simulink model "gui"  (R2012b)
settings: Solver=ode45  StartTime=0.0  StopTime=inf  RelTol=1e-3
undefined symbols (not defined in the file or in its folder): desired_torso_pitch, kd_lateral, kd_pitch, kd_sea_position, kd_sea_torque, ki_lateral, ki_sea_position, ki_sea_torque, kp_lateral, kp_pitch, kp_sea_position, kp_sea_torque, umich_kd1, umich_kd2, umich_kp1, umich_kp2, umich_sat_val1, umich_scuff1, umich_scuff2
libraries: simulink x20, xpclib x18
settings Model: Creator=wmartin  LastModifiedBy=wmartin

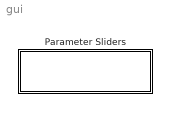
== system gui ==
  Parameter Sliders : Subsystem

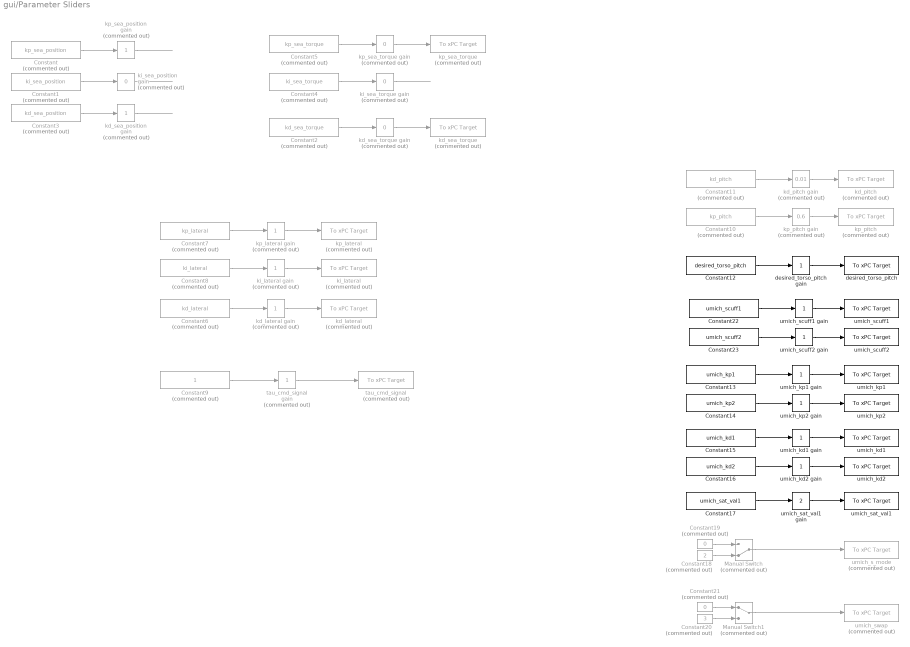
== system gui/Parameter Sliders ==
  Constant : Constant  Commented=on  Value=kp_sea_position
  Constant1 : Constant  Commented=on  Value=ki_sea_position
  Constant10 : Constant  Commented=on  Value=kp_pitch
  Constant11 : Constant  Commented=on  Value=kd_pitch
  Constant12 : Constant  Value=desired_torso_pitch
  Constant13 : Constant  Value=umich_kp1
  Constant14 : Constant  Value=umich_kp2
  Constant15 : Constant  Value=umich_kd1
  Constant16 : Constant  Value=umich_kd2
  Constant17 : Constant  Value=umich_sat_val1
  Constant18 : Constant  Commented=on  Value=2
  Constant19 : Constant  Commented=on  Value=0
  Constant2 : Constant  Commented=on  Value=kd_sea_torque
  Constant20 : Constant  Commented=on  Value=3
  Constant21 : Constant  Commented=on  Value=0
  Constant22 : Constant  Value=umich_scuff1
  Constant23 : Constant  Value=umich_scuff2
  Constant3 : Constant  Commented=on  Value=kd_sea_position
  Constant4 : Constant  Commented=on  Value=ki_sea_torque
  Constant5 : Constant  Commented=on  Value=kp_sea_torque
  Constant6 : Constant  Commented=on  Value=kd_lateral
  Constant7 : Constant  Commented=on  Value=kp_lateral
  Constant8 : Constant  Commented=on  Value=ki_lateral
  Constant9 : Constant  Commented=on
  Manual Switch : ManualSwitch  Commented=on  CurrentSetting=0
  Manual Switch1 : ManualSwitch  Commented=on
  desired_torso_pitch : xpclib/Misc./To xPC Target   appname=umich_2d_walking  blockpath=UMich Controller/desired_pitch  paramname=Value  isdefault=on
  desired_torso_pitch gain : simulink/Math Operations/Slider Gain  low=-10  gain=1  high=20
  kd_lateral : xpclib/Misc./To xPC Target   Commented=on  appname=umich_2d_walking  blockpath=UMich Controller/lateral_PID_control/Lateral Hip PID/Proportional Gain1  paramname=Gain  isdefault=on
  kd_lateral gain : simulink/Math Operations/Slider Gain  Commented=on  low=0  gain=1  high=5
  kd_pitch : xpclib/Misc./To xPC Target   Commented=on  appname=umich_2d_walking  blockpath=UMich Controller/Subsystem/Proportional Gain2  paramname=Gain  isdefault=on
  kd_pitch gain : simulink/Math Operations/Slider Gain  Commented=on  low=0  gain=0.01  high=0.1
  kd_sea_position gain : simulink/Math Operations/Slider Gain  Commented=on  low=0  gain=1  high=5
  kd_sea_torque : xpclib/Misc./To xPC Target   Commented=on  appname=umich_2d_walking  blockpath=Actuator Control/SEA Controller (Position)/kd_gain  paramname=Gain  isdefault=on
  kd_sea_torque gain : simulink/Math Operations/Slider Gain  Commented=on  low=0  gain=0  high=5
  ki_lateral : xpclib/Misc./To xPC Target   Commented=on  appname=umich_2d_walking  blockpath=UMich Controller/lateral_PID_control/Lateral Hip PID/Proportional Gain2  paramname=Gain  isdefault=on
  ki_lateral gain : simulink/Math Operations/Slider Gain  Commented=on  low=0  gain=1  high=5
  ki_sea_position gain : simulink/Math Operations/Slider Gain  Commented=on  low=0  gain=0  high=5
  ki_sea_torque gain : simulink/Math Operations/Slider Gain  Commented=on  low=0  gain=0  high=5
  kp_lateral : xpclib/Misc./To xPC Target   Commented=on  appname=umich_2d_walking  blockpath=UMich Controller/lateral_PID_control/Lateral Hip PID/Proportional Gain  paramname=Gain  isdefault=on
  kp_lateral gain : simulink/Math Operations/Slider Gain  Commented=on  low=0  gain=1  high=10
  kp_pitch : xpclib/Misc./To xPC Target   Commented=on  appname=umich_2d_walking  blockpath=UMich Controller/Subsystem/Proportional Gain1  paramname=Gain  isdefault=on
  kp_pitch gain : simulink/Math Operations/Slider Gain  Commented=on  low=0  gain=0.6  high=2
  kp_sea_position gain : simulink/Math Operations/Slider Gain  Commented=on  low=0  gain=1  high=5
  kp_sea_torque : xpclib/Misc./To xPC Target   Commented=on  appname=umich_2d_walking  blockpath=Actuator Control/SEA Controller (Position)/kp_gain  paramname=Value  isdefault=on
  kp_sea_torque gain : simulink/Math Operations/Slider Gain  Commented=on  low=0  gain=0  high=10
  tau_cmd_signal : xpclib/Misc./To xPC Target   Commented=on  appname=umich_2d_walking  blockpath=Actuator Control/tau_cmd_signal  paramname=Gain  isdefault=on
  tau_cmd_signal gain : simulink/Math Operations/Slider Gain  Commented=on  low=0  gain=1  high=5
  umich_kd1 : xpclib/Misc./To xPC Target   appname=umich_2d_walking  blockpath=UMich Controller/kd1  paramname=Value  isdefault=on
  umich_kd1 gain : simulink/Math Operations/Slider Gain  low=0  gain=1  high=200
  umich_kd2 : xpclib/Misc./To xPC Target   appname=umich_2d_walking  blockpath=UMich Controller/kd2  paramname=Value  isdefault=on
  umich_kd2 gain : simulink/Math Operations/Slider Gain  low=0  gain=1  high=200
  umich_kp1 : xpclib/Misc./To xPC Target   appname=umich_2d_walking  blockpath=UMich Controller/kp1  paramname=Value  isdefault=on
  umich_kp1 gain : simulink/Math Operations/Slider Gain  low=0  gain=1  high=200
  umich_kp2 : xpclib/Misc./To xPC Target   appname=umich_2d_walking  blockpath=UMich Controller/kp2  paramname=Value  isdefault=on
  umich_kp2 gain : simulink/Math Operations/Slider Gain  low=0  gain=1  high=200
  umich_s_mode : xpclib/Misc./To xPC Target   Commented=on  appname=umich_2d_walking  blockpath=UMich Controller/s_mode  paramname=Value  isdefault=on
  umich_sat_val1 : xpclib/Misc./To xPC Target   appname=umich_2d_walking  blockpath=UMich Controller/sat_val1  paramname=Value  isdefault=on
  umich_sat_val1 gain : simulink/Math Operations/Slider Gain  low=0  gain=2  high=4
  umich_scuff1 : xpclib/Misc./To xPC Target   appname=umich_2d_walking  blockpath=UMich Controller/scuff1  paramname=Value  isdefault=on
  umich_scuff1 gain : simulink/Math Operations/Slider Gain  low=0  gain=1  high=40
  umich_scuff2 : xpclib/Misc./To xPC Target   appname=umich_2d_walking  blockpath=UMich Controller/scuff2  paramname=Value  isdefault=on
  umich_scuff2 gain : simulink/Math Operations/Slider Gain  low=0  gain=1  high=40
  umich_swap : xpclib/Misc./To xPC Target   Commented=on  appname=umich_2d_walking  blockpath=UMich Controller/swap  paramname=Value  isdefault=on
  wires:
  kp_sea_position gain/1 -> ?
  Constant/1 -> kp_sea_position gain/1
  Constant1/1 -> ki_sea_position gain/1
  ki_sea_position gain/1 -> ?
  Constant3/1 -> kd_sea_position gain/1
  kd_sea_position gain/1 -> ?
  ki_sea_torque gain/1 -> ?
  Constant4/1 -> ki_sea_torque gain/1
  Constant5/1 -> kp_sea_torque gain/1
  kp_sea_torque gain/1 -> kp_sea_torque/1
  Constant6/1 -> kd_lateral gain/1
  Constant7/1 -> kp_lateral gain/1
  Constant8/1 -> ki_lateral gain/1
  kd_lateral gain/1 -> kd_lateral/1
  ki_lateral gain/1 -> ki_lateral/1
  kp_lateral gain/1 -> kp_lateral/1
  Constant2/1 -> kd_sea_torque gain/1
  kd_sea_torque gain/1 -> kd_sea_torque/1
  tau_cmd_signal gain/1 -> tau_cmd_signal/1
  Constant9/1 -> tau_cmd_signal gain/1
  Constant10/1 -> kp_pitch gain/1
  Constant11/1 -> kd_pitch gain/1
  kd_pitch gain/1 -> kd_pitch/1
  kp_pitch gain/1 -> kp_pitch/1
  Constant12/1 -> desired_torso_pitch gain/1
  desired_torso_pitch gain/1 -> desired_torso_pitch/1
  Constant13/1 -> umich_kp1 gain/1
  umich_kp1 gain/1 -> umich_kp1/1
  Constant14/1 -> umich_kp2 gain/1
  Constant15/1 -> umich_kd1 gain/1
  Constant16/1 -> umich_kd2 gain/1
  Constant17/1 -> umich_sat_val1 gain/1
  umich_kp2 gain/1 -> umich_kp2/1
  umich_kd1 gain/1 -> umich_kd1/1
  umich_kd2 gain/1 -> umich_kd2/1
  umich_sat_val1 gain/1 -> umich_sat_val1/1
  Constant18/1 -> Manual Switch/2
  Constant19/1 -> Manual Switch/1
  Constant20/1 -> Manual Switch1/2
  Constant21/1 -> Manual Switch1/1
  Manual Switch/1 -> umich_s_mode/1
  Manual Switch1/1 -> umich_swap/1
  Constant22/1 -> umich_scuff1 gain/1
  umich_scuff1 gain/1 -> umich_scuff1/1
  Constant23/1 -> umich_scuff2 gain/1
  umich_scuff2 gain/1 -> umich_scuff2/1
